simulink model "cl_PWM"  (R2023a)
settings: Solver=FixedStepDiscrete  StartTime=0.0  StopTime=.35  FixedStep=Ts  RelTol=1e-3  EnableMultiTasking=on
PreLoadFcn:
  | ee_ipmsm_velocity_control_data;
StopFcn:
  | ee_addSimlogTimeStamp(bdroot)
values from neighbouring files (symbols this model uses):
  ActCV = 1    [cl_PWM_Parameter.m]
  ActFF = 0    [cl_PWM_Parameter.m]
  down1 = den(1)    [cl_PWM_Parameter.m]
  down2 = den(2)    [cl_PWM_Parameter.m]
  Jm = 7.0616e-06    [cl_PWM_Parameter.m]
  Ki_iq = Ki_id    (= 173.2)    [cl_PWM_Parameter.m]
  Kp_id = 0.6*Tl/Vs/sigma    (= 0.0866)    [cl_PWM_Parameter.m]
  Kp_iq = Kp_id    (= 0.0866)    [cl_PWM_Parameter.m]
  Ld = 0.2e-3    (= 0.0002)    [cl_PWM_Parameter.m]
  Lq = 0.2e-3    (= 0.0002)    [cl_PWM_Parameter.m]
  p = 4    [cl_PWM_Parameter.m]
  psim = 0.0064    [cl_PWM_Parameter.m]
  Trated = 0.2724    [cl_PWM_Parameter.m]
  Ts = 1e-6    (= 1e-06)    [cl_PWM_Parameter.m]
  Tsi = 1/fsw/2    (= 0.0001)    [cl_PWM_Parameter.m]
  Tso = 2*Tsi    (= 0.0002)    [cl_PWM_Parameter.m]
  up = num(2)    [cl_PWM_Parameter.m]
  Vnom = 24    [cl_PWM_Parameter.m]
undefined symbols (not defined in the file or in its folder): denZC_id, denZC_iq, ee_sli_rtmsupport, gcbh, numZC_id, numZC_iq
libraries: nesl_utility x15, fl_lib x10, slpidlib x9, ee_lib x7, spsMeanLib x6, simulink x3, eeTransforms x2, SignalEditorBlockLib x1, eePwmGeneratorTwoLevel x1, slctrlblks x1
(part 1 of 2)
CloseFcn:
  | try,close(h1_ee_ipmsm_velocity_control),end
  | clear h1_ee_ipmsm_velocity_control
  | 
  | clear simlog_ee_ipmsm_velocity_control
  | clear logsout_ee_ipmsm_velocity_control
  | 
  | clear Pmax Tmax p psim Ld Lq L0 Rs Jm
  | clear Cdc Vnom V1 AH0
  | clear Ts fsw Tsi Tso Kp_id Ki_id Kp_iq Ki_iq
  | clear numd_id dend_id numd_iq dend_iq
  | clear Kp_omega Ki_omega numd_omega dend_omega
  | clear ID_MAP IQ_MAP RPM_VECT TQ_VECT VDC_VECT
Description:
  | IPMSM Velocity Control
settings Model: SimulationMode=accelerator  Creator=The MathWorks, Inc.  LastModifiedBy=zxzhu
settings SolverCC: AlgebraicLoopSolver=TrustRegion  AutoInsertRateTranBlk=on  MaxZcPerStep=1
settings DataIOCC: MaxDataPoints=210000  ReturnWorkspaceOutputs=off  SignalLoggingName=logsout_ee_ipmsm_velocity_control
settings OptimizationCC: ReuseModelBlockBuffer=off  LifeSpan=inf
settings DebuggingCC: UnderspecifiedInitializationDetection=Classic  MergeDetectMultiDrivingBlocksExec=none  UnconnectedInputMsg=warning  UnconnectedOutputMsg=warning  UnconnectedLineMsg=warning  SFUnexpectedBacktrackingDiag=warning  SFNoUnconditionalDefaultTransitionDiag=warning  SFExecutionAtInitializationDiag=none  ArithmeticOperatorsInVariantConditions=warning
settings ModelReferenceCC: EnableRefExpFcnMdlSchedulingChecks=on
settings SFSimCC: SimUseLocalCustomCode=off  CustomCodeUndefinedFunction=UseInterfaceOnly
settings RTWCC: RTWUseLocalCustomCode=off  DLArmComputeVersion=19.05
settings CodeAppCC: StateflowObjectComments=on
settings GRTTargetCC: TargetLangStandard=C89/C90 (ANSI)
settings ConfigComp: CovMetricSettings=dw  CovSaveCumulativeToWorkspaceVar=on  CovSaveSingleToWorkspaceVar=on  CovExternalEMLEnable=off
settings SimscapeCC: SimscapeNormalizeSystem=off  SimscapeLogType=all  SimscapeLogSimulationStatistics=on  SimscapeLogName=simlog_ee_ipmsm_velocity_control  SimscapeLogDataHistory=210000

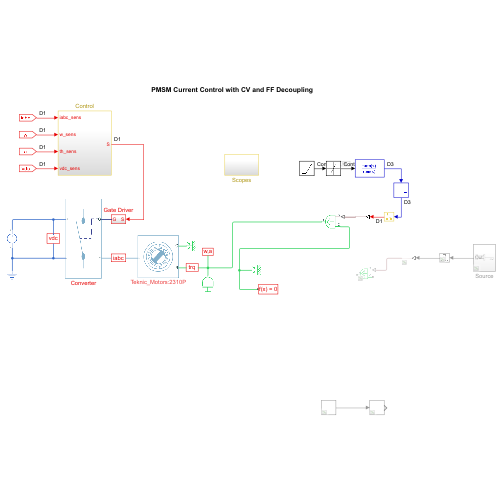
[thumbnail: Simulink's stored preview of the top-level diagram]
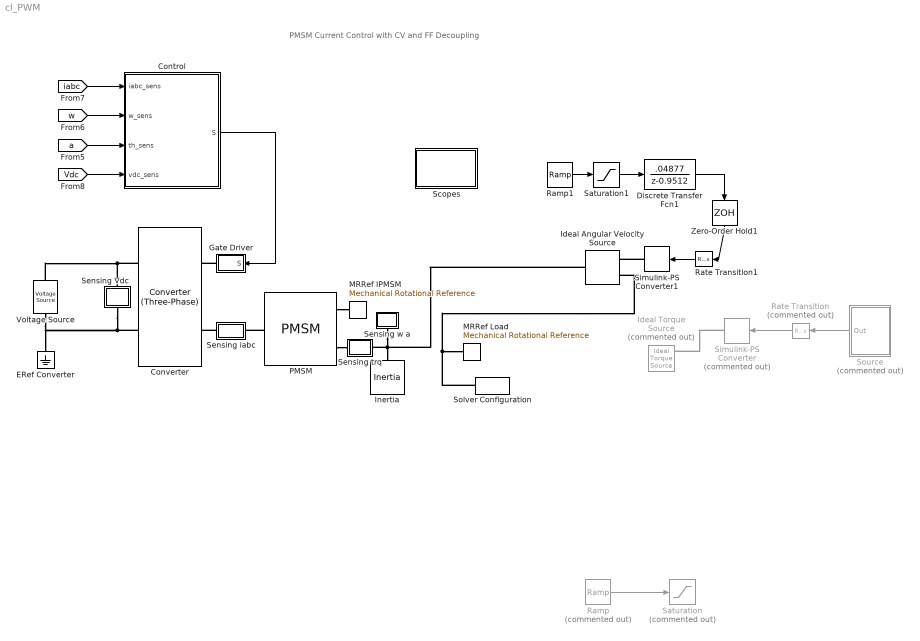
== system cl_PWM ==
  note: PMSM Current Control with CV and FF Decoupling
  Control : Subsystem
  Converter : ee_lib/Semiconductors & Converters/Converters/Converter (Three-Phase)  port_option=ee.enum.threePhasePort.composite  device_type=ee.enum.converters.switchingdevice.mosfet  K=0  Vf=0.8 V  Ron=0.001 Ohm  Rds=0.001 Ohm  Goff=1e-5 1/Ohm  Vgt=1 V  Vgt_off=-1 V  Ih=1 A  Vth=0.5 V  diode_param=2  diode_Vf=0.8 V  diode_Ron=0.001 Ohm  diode_Goff=1e-5 1/Ohm  diode_C=50 nF  diode_iRM=-235 A  diode_iF=300 A  diode_idot=-50 A/us  diode_trr_param=1  diode_trr_factor=3  diode_trr=15 us  diode_Qrr=1.5e+3 s*uA  snubber_type=ee.enum.converters.snubber.include  Cs=1e-7 F  Rs=0.1 Ohm
  Discrete Transfer Fcn1 : DiscreteTransferFcn  Numerator=[.04877]  Denominator=[1 -0.9512]  SampleTime=Tsi
  ERef Converter : fl_lib/Electrical/Electrical Elements/Electrical Reference
  Gate Driver : Subsystem
  Ideal Angular Velocity Source : fl_lib/Mechanical/Mechanical Sources/Ideal Angular Velocity Source
  Ideal Torque Source : fl_lib/Mechanical/Mechanical Sources/Ideal Torque Source  Commented=on
  Inertia : fl_lib/Mechanical/Rotational Elements/Inertia  inertia=Jm kg*m^2  num_ports=foundation.enum.numPorts2.one  w_specify=on  w_priority=High  w=0 rpm  w_nominal_specify=off  w_nominal_unit=rad/s  w_nominal_value=1  t_specify=off  t_priority=High  t=0 N*m  t_nominal_specify=off  t_nominal_unit=N*m  t_nominal_value=1
  MRRef IPMSM : fl_lib/Mechanical/Rotational Elements/Mechanical Rotational Reference
  MRRef Load : fl_lib/Mechanical/Rotational Elements/Mechanical Rotational Reference
  PMSM : ee_lib/Electromechanical/Permanent Magnet/PMSM  Tag={'toolbox/physmod/elec/library/m/ee_lib_parts';'Electromechanical/Permanent_Magnet/PMSM/Teknic_Motors/x2310P.xml'}  port_option=ee.enum.threePhasePort.composite  winding_type=ee.enum.statorconnection.wye  machine_param=ee.enum.pmsm.parameterization.constant  nPolePairs=p  pmflux_param=ee.enum.pmflux.fluxlinkage  pm_flux_linkage=psim Wb  torque_constant=0.0255816607475711 N*m/A  back_emf_constant=0.0255816607475711 V/(rad/s)  stator_param=ee.enum.statorparam.LdLqL0  Ld=Ld H  Lq=Lq H  idVec=[-200 0 200] % Parameter not set A  iqVec=[-200 0 200] % Parameter not set A  LdMatrix=[0.0002 0.0002 0.0002;0.0002 0.0002 0.0002;0.0002 0.0002 0.0002] % Parameter not set H  LqMatrix=[0.0002 0.0002 0.0002;0.0002 0.0002 0.0002;0.0002 0.0002 0.0002] % Parameter not set H  PmMatrix=[0.1 0.1 0.1;0.1 0.1 0.1;0.1 0.1 0.1] Wb  ktMatrix=[0.18 0.18 0.18;0.18 0.18 0.18;0.18 0.18 0.18] N*m/A  keMatrix=[0.18 0.18 0.18;0.18 0.18 0.18;0.18 0.18 0.18] % Parameter not set V/(rad/s)  L0=[] % Parameter not set H  Ls=0.0002 H  Lm=-2e-05 H  Ms=2e-05 H  Rs=Rs Ohm  zero_sequence=ee.enum.park.zerosequence.exclude  axes_param=ee.enum.rotorangle.daxis  loss_param=ee.enum.ironloss.none  losses_oc=[0 0 0] % Parameter not set W  losses_sc=[0 0 0] % Parameter not set W  f_losses=60 % Parameter not set Hz  Isc_losses=95 % Parameter not set A  J=Jm kg*m^2  lam=Trated*.01/3000*9.55 N*m/(rad/s)  i_d_specify=off  i_d_priority=None  i_d=0 A  i_d_nominal_specify=off  i_d_nominal_unit=A  i_d_nominal_value=1  i_q_specify=off  i_q_priority=None  i_q=0 A  i_q_nominal_specify=off  i_q_nominal_unit=A  i_q_nominal_value=1  torque_specify=off  torque_priority=None  torque=0 N*m  torque_nominal_specify=off  torque_nominal_unit=N*m  torque_nominal_value=1  angular_velocity_specify=off  angular_velocity_priority=None  angular_velocity=0 rpm  angular_velocity_nominal_specify=off  angular_velocity_nominal_unit=rpm  angular_velocity_nominal_value=1  angular_position_specify=off  angular_position_priority=High  angular_position=0 rad  angular_position_nominal_specify=off  angular_position_nominal_unit=deg  angular_position_nominal_value=1  alpha=3.93e-3 1/K  alpha_flux=-0.001 1/K  Tmeas=298.15 K  stator_thermal_mass=100 J/K  rotor_thermal_mass=200 J/K  Rm_percent_rotor=90  Rd_percent_rotor=30  temperatureA_specify=off  temperatureA_priority=High  temperatureA=25 degC  temperatureA_nominal_specify=off  temperatureA_nominal_unit=degC  temperatureA_nominal_value=1  temperatureB_specify=off  temperatureB_priority=High  temperatureB=25 degC  temperatureB_nominal_specify=off  temperatureB_nominal_unit=degC  temperatureB_nominal_value=1  temperatureC_specify=off  temperatureC_priority=High  temperatureC=25 degC  temperatureC_nominal_specify=off  temperatureC_nominal_unit=degC  temperatureC_nominal_value=1  temperatureR_specify=off  temperatureR_priority=High  temperatureR=25 degC  temperatureR_nominal_specify=off  temperatureR_nominal_unit=degC  temperatureR_nominal_value=1
      settings: AttributesFormatString=Teknic_Motors:2310P  InternalSimscapePortConfiguration="{\"Bottom\":[],\"Left\":[{\"id\":\"N\",\"label\":\"~\",\"type\":\"foundation.electrical.three_phase\"}],\"Right\":[{\"id\":\"R\",\"label\":\"R\",\"type\":\"foundation.mechanical.rotational.rotational\"},{\"id\":\"C\",\"label\":\"C\",\"type\":\"foundation.mechanical.rotational.rotational\"}],\"Top\":[]}"
  Ramp : simulink/Sources/Ramp  Commented=on  slope=-Trated/.001  start=.25  InitialOutput=0
  Ramp1 : simulink/Sources/Ramp  slope=-3000/9.55/.1  start=0  InitialOutput=0
  Rate Transition : RateTransition  Commented=on  OutPortSampleTime=Ts
  Rate Transition1 : RateTransition  OutPortSampleTime=Ts
  Saturation : Saturate  Commented=on  UpperLimit=.5*Trated  LowerLimit=-.5*Trated
  Saturation1 : Saturate  UpperLimit=3000/9.55*1  LowerLimit=-4800/9.55*1
  Scopes : Subsystem
  Sensing Vdc : Subsystem
      mask Display: disp('vdc')
  Sensing trq : Subsystem
      mask Display: disp('trq')
  Sensing w a : Subsystem
      mask Display: disp('w,a')
  Sensing iabc : Subsystem
      mask Display: disp('iabc')
  Simulink-PS Converter : nesl_utility/Simulink-PS Converter  Commented=on  PhysicalDomain=network_engine_domain  SubClassName=ps_input  LeftPortType=input  RightPortType=output  PseudoPeriodic=off  Frequencies=[]  NoiseDistribution=none  NoiseParameters=[]  Unit=N*m  AffineConversion=off  FilteringAndDerivatives=zero  SimscapeFilterOrder=1  InputFilterTimeConstant=0.001  UdotUserProvided=1
  Simulink-PS Converter1 : nesl_utility/Simulink-PS Converter  PhysicalDomain=network_engine_domain  SubClassName=ps_input  LeftPortType=input  RightPortType=output  PseudoPeriodic=off  Frequencies=[]  NoiseDistribution=none  NoiseParameters=[]  Unit=rad/s  AffineConversion=off  FilteringAndDerivatives=zero  SimscapeFilterOrder=1  InputFilterTimeConstant=0.001  UdotUserProvided=1
  Solver Configuration : nesl_utility/Solver Configuration  PhysicalDomain=network_engine_domain  SubClassName=solver  LeftPortType=input  RightPortType=generic  Tones=[]  Harmonics=[]  SimulateNoise=off  Profile=off  UseLocalSampling=off  EnableSwitchedLinearOptims=on  FrequencyDomain=off  UseCCode=off  RelTol=0.001  AbsTol=1e-06  MinStep=1e-09  ToWorkspace=off  RevertToSquareIcSolve=off  NumHomotopyIterations=100  PhasorMode=off  PhasorModeNumHarmonics=1  ConsistencySolver=NEWTON_FTOL  IndexReductionMethod=DerivativeReplacement  DoDC=off  ResidualTolerance=1e-9  ConsistencyTolSource=GLOBAL  ConsistencyAbsTol=0.001  ConsistencyRelTol=0.001  ConsistencyTolFactor=0.001  UseLocalSolver=on  LocalSolverChoice=NE_BACKWARD_EULER_ADVANCER  ResolveIndetEquations=on  FunctionEvalNumThread=1  LocalSolverSampleTime=Ts  DoFixedCost=on  MaxNonlinIter=5  MaxModeIter=2  ComputeImpulses=off  ImpulseIterations=2  LinearAlgebra=auto  LinearAlgebraNumThread=0  EquationFormulation=NE_TIME_EF  DelaysMemoryBudget=1024  AutomaticFiltering=on  FilteringTimeConstant=0.001  PartitionStorageMethod=AS_NEEDED  PartitionMemoryBudget=1024  PartitionMethod=FAST
  Source : Subsystem  Commented=on
  Voltage Source : ee_lib/Sources/Voltage Source  dc_voltage=Vnom V  ac_voltage=0 V  ac_shift=0 rad  ac_frequency=60 Hz  noise_mode=ee.enum.sources.noise.Disabled  PSD=0 V^2/Hz  sample_time=1e-3 s  repeatability=ee.enum.sources.repeatability.NotRepeatable  user_seed=0  auto_seed=3499211588  i_specify=off  i_priority=None  i=0 A  i_nominal_specify=off  i_nominal_unit=A  i_nominal_value=1  v_specify=off  v_priority=None  v=0 V  v_nominal_specify=off  v_nominal_unit=V  v_nominal_value=1
  Zero-Order Hold1 : ZeroOrderHold  SampleTime=-1
  wires:
  Control/1(S) -> Gate Driver/1(S)
  [Vdc] -> Control/4(vdc_sens)
  [iabc] -> Control/1(iabc_sens)
  [w] -> Control/2(w_sens)
  [a] -> Control/3(th_sens)
  Zero-Order Hold1/1 -> Rate Transition1/1
  Discrete Transfer Fcn1/1 -> Zero-Order Hold1/1
  Ramp1/1 -> Saturation1/1
  Saturation1/1 -> Discrete Transfer Fcn1/1
  Rate Transition1/1 -> Simulink-PS Converter1/1
  Ramp/1 -> Saturation/1
  Source/1(Out) -> Rate Transition/1
  Rate Transition/1 -> Simulink-PS Converter/1
  connections:
  Converter/RConn1 -- Voltage Source/LConn1 -- Sensing Vdc/LConn1
  Inertia/LConn1 -- Ideal Angular Velocity Source/LConn1 -- Sensing w a/LConn1 -- Sensing trq/RConn1
  Gate Driver/RConn1 -- Converter/LConn1
  Solver Configuration/RConn1 -- Ideal Angular Velocity Source/RConn2 -- MRRef Load/LConn1
  Sensing iabc/LConn1 -- Converter/LConn2
  PMSM/RConn2 -- MRRef IPMSM/LConn1
  PMSM/RConn1 -- Sensing trq/LConn1
  Voltage Source/RConn1 -- ERef Converter/LConn1 -- Converter/RConn2 -- Sensing Vdc/RConn1
  PMSM/LConn1 -- Sensing iabc/RConn1
  Simulink-PS Converter1/RConn1 -- Ideal Angular Velocity Source/RConn1
  Simulink-PS Converter/RConn1 -- Ideal Torque Source/RConn1

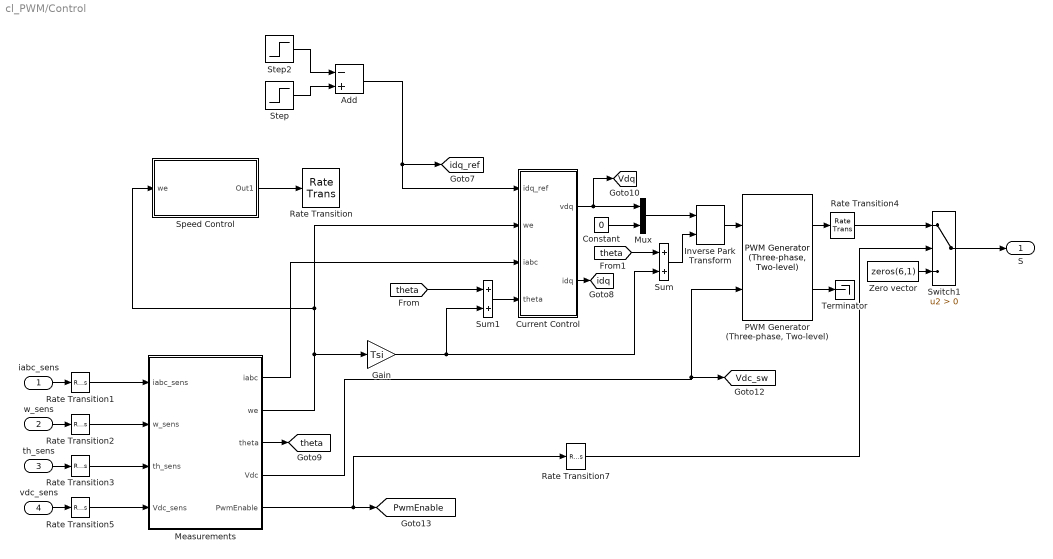
== system cl_PWM/Control ==
  iabc_sens : Inport
  w_sens : Inport  Port=2
  th_sens : Inport  Port=3
  vdc_sens : Inport  Port=4
  Add : Sum  Inputs=-+
  Constant : Constant  Value=0  SampleTime=Tsi
  Current Control : Subsystem
  Gain : Gain  Gain=Tsi
  Inverse Park Transform : eeTransforms/Inverse Park Transform  AxisAlignment=D-axis  PowerInvariant=off
  Measurements : Subsystem
  Mux : Mux  Inputs=2
  "PWM Generator (Three-phase, Two-level)" : eePwmGeneratorTwoLevel/PWM Generator (Three-phase, Two-level)  PWMMode=Continuous PWM (CPWM)  CPWMMode=SVM: space vector modulation  DPWMMode=60 DPWM: 60 degree discontinuous PWM  fsw=fsw  Ts=Ts
      settings: SamplingMode=Asymmetric
  Rate Transition : RateTransition  OutPortSampleTime=Tsi
  Rate Transition{1..3,5,7} (5 alike) : RateTransition
  Rate Transition4 : RateTransition  OutPortSampleTime=Ts
  Speed Control : Subsystem
  Step : Step  Time=.2  Before=[0 0]  After=[0 0.71]  SampleTime=Tsi
  Step2 : Step  Time=.25  Before=[0 0]  After=[0 0.3]  SampleTime=Tsi
  Sum : Sum
  Sum1 : Sum
  Switch1 : Switch  Criteria=u2 > Threshold  SaturateOnIntegerOverflow=off  InputSameDT=off
  Terminator : Terminator
  Zero vector : Constant  Value=zeros(6,1)
  S : Outport  VectorParamsAs1DForOutWhenUnconnected=off
  tag scope: PwmEnable=global, Vdc_sw=global, Vdq=global, idq=global, idq_ref=global, theta=global
  wires:
  Current Control/1(vdq) -> Mux/1, [Vdq]
  Measurements/1(iabc) -> Current Control/3(iabc)
  "PWM Generator (Three-phase, Two-level)"/1 -> Rate Transition4/1
  iabc_sens/1 -> Rate Transition1/1
  w_sens/1 -> Rate Transition2/1
  th_sens/1 -> Rate Transition3/1
  vdc_sens/1 -> Rate Transition5/1
  "PWM Generator (Three-phase, Two-level)"/2 -> Terminator/1
  Rate Transition1/1 -> Measurements/1(iabc_sens)
  Rate Transition2/1 -> Measurements/2(w_sens)
  Rate Transition3/1 -> Measurements/3(th_sens)
  Rate Transition5/1 -> Measurements/4(Vdc_sens)
  Measurements/4(Vdc) -> "PWM Generator (Three-phase, Two-level)"/2, [Vdc_sw]
  Measurements/2(we) -> Gain/1, Speed Control/1(we), Current Control/2(we)
  Current Control/2(idq) -> [idq]
  Switch1/1 -> S/1
  Rate Transition4/1 -> Switch1/1
  Measurements/5(PwmEnable) -> Rate Transition7/1, [PwmEnable]
  Zero vector/1 -> Switch1/3
  Rate Transition7/1 -> Switch1/2
  Constant/1 -> Mux/2
  Inverse Park Transform/1 -> "PWM Generator (Three-phase, Two-level)"/1
  Mux/1 -> Inverse Park Transform/1
  Measurements/3(theta) -> [theta]
  [theta] -> Sum/1
  Sum/1 -> Inverse Park Transform/2
  Gain/1 -> Sum1/2, Sum/2
  Sum1/1 -> Current Control/4(theta)
  [theta] -> Sum1/1
  Speed Control/1(Out1) -> Rate Transition/1
  Step2/1 -> Add/1
  Step/1 -> Add/2
  Add/1 -> Current Control/1(idq_ref), [idq_ref]

== system cl_PWM/Gate Driver ==
  S : Inport
  Demux : Demux  Outputs=6
  Simulink-PS Converter{1..6} (6 alike) : nesl_utility/Simulink-PS Converter  PhysicalDomain=network_engine_domain  SubClassName=ps_input  LeftPortType=input  RightPortType=output  PseudoPeriodic=off  Frequencies=[]  NoiseDistribution=none  NoiseParameters=[]  Unit=1  AffineConversion=off  FilteringAndDerivatives=zero  SimscapeFilterOrder=1  InputFilterTimeConstant=0.001  UdotUserProvided=1
  Six-Pulse Gate Multiplexer : ee_lib/Semiconductors & Converters/Converters/Six-Pulse Gate Multiplexer  port_option=ee.enum.controlport.ps
  G : PMIOPort  Side=Right
  wires:
  Demux/1 -> Simulink-PS Converter1/1
  S/1 -> Demux/1
  Demux/4 -> Simulink-PS Converter4/1
  Demux/2 -> Simulink-PS Converter2/1
  Demux/3 -> Simulink-PS Converter3/1
  Demux/5 -> Simulink-PS Converter5/1
  Demux/6 -> Simulink-PS Converter6/1
  connections:
  Six-Pulse Gate Multiplexer/RConn1 -- G/RConn1
  Simulink-PS Converter1/RConn1 -- Six-Pulse Gate Multiplexer/LConn1
  Simulink-PS Converter3/RConn1 -- Six-Pulse Gate Multiplexer/LConn3
  Simulink-PS Converter5/RConn1 -- Six-Pulse Gate Multiplexer/LConn5
  Simulink-PS Converter6/RConn1 -- Six-Pulse Gate Multiplexer/LConn6
  Simulink-PS Converter4/RConn1 -- Six-Pulse Gate Multiplexer/LConn4
  Simulink-PS Converter2/RConn1 -- Six-Pulse Gate Multiplexer/LConn2

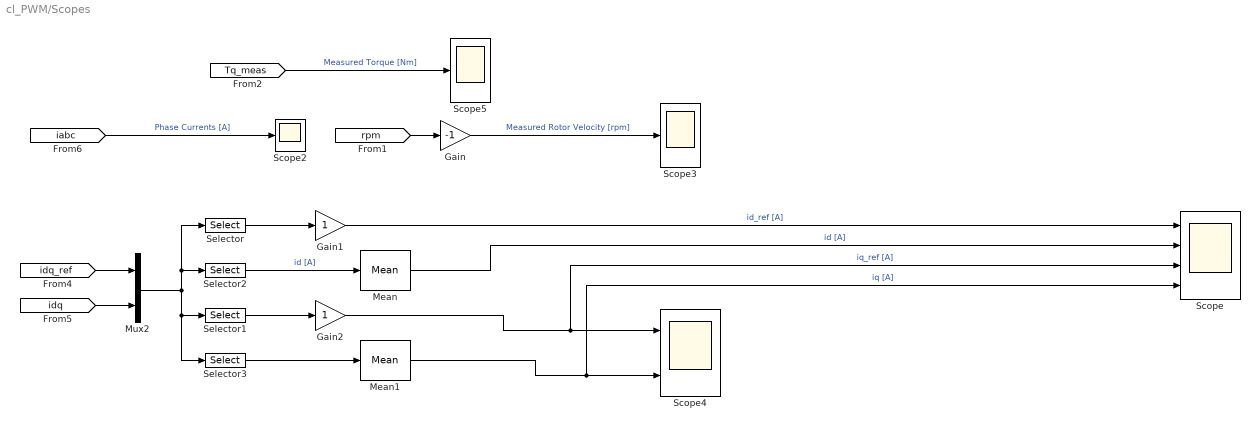
== system cl_PWM/Scopes ==
  Gain : Gain  Gain=-1
  Gain1 : Gain
  Gain2 : Gain
  Mean : spsMeanLib/Mean  Freq=1/Tsi  Vinit=0  Ts=Ts
  Mean1 : spsMeanLib/Mean  Freq=1/Tsi  Vinit=0  Ts=Ts
  Mux2 : Mux  Inputs=2
  Scope : Scope  NumInputPorts=4
  Scope2 : Scope
  Scope3 : Scope
  Scope4 : Scope  NumInputPorts=2
  Scope5 : Scope
  Selector : Selector  InputPortWidth=4  IndexOptions=Index vector (dialog)  Indices=1  OutputSizes=1
  Selector1 : Selector  InputPortWidth=4  IndexOptions=Index vector (dialog)  Indices=2  OutputSizes=1
  Selector2 : Selector  InputPortWidth=4  IndexOptions=Index vector (dialog)  Indices=3  OutputSizes=1
  Selector3 : Selector  InputPortWidth=4  IndexOptions=Index vector (dialog)  Indices=4  OutputSizes=1
  wires:
  Mux2/1 -> Selector3/1, Selector1/1, Selector2/1, Selector/1
  [idq_ref] -> Mux2/1
  [iabc] -> Scope2/1  "Phase Currents [A]"
  [idq] -> Mux2/2
  Selector/1 -> Gain1/1
  Selector1/1 -> Gain2/1
  Gain1/1 -> Scope/1  "id_ref [A]"
  Gain2/1 -> Scope/3, Scope4/1  "iq_ref [A]"
  Mean/1 -> Scope/2  "id [A]"
  [Tq_meas] -> Scope5/1  "Measured Torque [Nm]"
  Selector3/1 -> Mean1/1
  Gain/1 -> Scope3/1  "Measured Rotor Velocity [rpm]"
  Selector2/1 -> Mean/1  "id [A]"
  Mean1/1 -> Scope/4, Scope4/2  "iq [A]"
  [rpm] -> Gain/1

== system cl_PWM/Sensing Vdc ==
  PS-Simulink Converter4 : nesl_utility/PS-Simulink Converter  PhysicalDomain=network_engine_domain  SubClassName=ps_output  LeftPortType=input  RightPortType=output  PseudoPeriodic=off  Frequencies=[]  VectorFormat=1-D array  Unit=V  AffineConversion=off
  Voltage Sensor : fl_lib/Electrical/Electrical Sensors/Voltage Sensor
  + : PMIOPort  Side=Left
  - : PMIOPort  Port=2  Side=Right
  tag scope: Vdc=global
  wires:
  PS-Simulink Converter4/1 -> [Vdc]
  connections:
  Voltage Sensor/LConn1 -- +/RConn1
  Voltage Sensor/RConn2 -- -/RConn1
  PS-Simulink Converter4/LConn1 -- Voltage Sensor/RConn1

== system cl_PWM/Sensing trq ==
  PS-Simulink Converter3 : nesl_utility/PS-Simulink Converter  PhysicalDomain=network_engine_domain  SubClassName=ps_output  LeftPortType=input  RightPortType=output  PseudoPeriodic=off  Frequencies=[]  VectorFormat=1-D array  Unit=N*m  AffineConversion=off
  Torque Sensor : fl_lib/Mechanical/Mechanical Sensors/Ideal Torque Sensor
  R : PMIOPort  Side=Left
  C : PMIOPort  Port=2  Side=Right
  tag scope: Tq_meas=global
  wires:
  PS-Simulink Converter3/1 -> [Tq_meas]
  connections:
  Torque Sensor/RConn1 -- C/RConn1
  Torque Sensor/RConn2 -- PS-Simulink Converter3/LConn1
  Torque Sensor/LConn1 -- R/RConn1

== system cl_PWM/Sensing w a ==
  MRRef : fl_lib/Mechanical/Rotational Elements/Mechanical Rotational Reference
  Motion Sensor : fl_lib/Mechanical/Mechanical Sensors/Ideal Rotational Motion Sensor  reference=foundation.enum.MeasurementReference.difference  acceleration_port=false  velocity_port=true  position_port=true  wrap_angle=false  offset=0 rad
  PS-Simulink Converter1 : nesl_utility/PS-Simulink Converter  PhysicalDomain=network_engine_domain  SubClassName=ps_output  LeftPortType=input  RightPortType=output  PseudoPeriodic=off  Frequencies=[]  VectorFormat=1-D array  Unit=rad/s  AffineConversion=off
  PS-Simulink Converter2 : nesl_utility/PS-Simulink Converter  PhysicalDomain=network_engine_domain  SubClassName=ps_output  LeftPortType=input  RightPortType=output  PseudoPeriodic=off  Frequencies=[]  VectorFormat=1-D array  Unit=rad  AffineConversion=off
  Rate Transition : RateTransition  OutPortSampleTime=Ts
  R : PMIOPort  Side=Left
  tag scope: a=global, w=global
  wires:
  PS-Simulink Converter1/1 -> [w]
  PS-Simulink Converter2/1 -> Rate Transition/1
  Rate Transition/1 -> [a]
  connections:
  R/RConn1 -- Motion Sensor/LConn1
  Motion Sensor/RConn2 -- PS-Simulink Converter1/LConn1
  MRRef/LConn1 -- Motion Sensor/RConn1
  PS-Simulink Converter2/LConn1 -- Motion Sensor/RConn3

== system cl_PWM/Sensing iabc ==
  Current Sensor : ee_lib/Sensors & Transducers/Current Sensor (Three-Phase)
  Floating Neutral (Three-Phase) : ee_lib/Connectors & References/Floating Neutral (Three-Phase)  G_parasitic=1e-12 1/Ohm
      settings: InternalSimscapePortConfiguration="{\"Bottom\":[],\"Left\":[{\"id\":\"N\",\"label\":\"~\",\"type\":\"foundation.electrical.three_phase\"}],\"Right\":[],\"Top\":[]}"
  PS-Simulink Converter : nesl_utility/PS-Simulink Converter  PhysicalDomain=network_engine_domain  SubClassName=ps_output  LeftPortType=input  RightPortType=output  PseudoPeriodic=off  Frequencies=[]  VectorFormat=1-D array  Unit=A  AffineConversion=off
  PS-Simulink Converter1 : nesl_utility/PS-Simulink Converter  PhysicalDomain=network_engine_domain  SubClassName=ps_output  LeftPortType=input  RightPortType=output  PseudoPeriodic=off  Frequencies=[]  VectorFormat=1-D array  Unit=V  AffineConversion=off
  Phase Voltage Sensor (Three-Phase) : ee_lib/Sensors & Transducers/Phase Voltage Sensor (Three-Phase)
  1 : PMIOPort  Side=Left
  2 : PMIOPort  Port=2  Side=Right
  tag scope: Vline=global, iabc=global
  wires:
  PS-Simulink Converter/1 -> [iabc]
  PS-Simulink Converter1/1 -> [Vline]
  connections:
  1/RConn1 -- Current Sensor/LConn1 -- Phase Voltage Sensor (Three-Phase)/LConn1
  2/RConn1 -- Current Sensor/RConn2
  Current Sensor/RConn1 -- PS-Simulink Converter/LConn1
  Floating Neutral (Three-Phase)/LConn1 -- Phase Voltage Sensor (Three-Phase)/RConn2
  PS-Simulink Converter1/LConn1 -- Phase Voltage Sensor (Three-Phase)/RConn1

== system cl_PWM/Source ==
  Add2 : Sum  Inputs=-+
  Step2 : Step  Time=.2  After=Trated*0.5  SampleTime=Tsi
  Step3 : Step  Time=.25  After=Trated*0.5  SampleTime=Tsi
  Out : Outport
  wires:
  Step2/1 -> Add2/2
  Step3/1 -> Add2/1
  Add2/1 -> Out/1

== system cl_PWM/Control/Current Control ==
  idq_ref : Inport
  we : Inport  Port=2
  iabc : Inport  Port=3
  theta : Inport  Port=4
  Constant : Constant  Value=0  SampleTime=Tsi
  PMSM Current Controller with Pre-Control and CV Decoupling : Subsystem  Commented=on  AncestorBlock=eePmsmCurrentController/PMSM Current Controller with Pre-Control  LoadFcn=ee_sli_rtmsupport( 'loadfcn', gcbh );  mask(PMSM Current Controller with Pre-Control){Kp_id=Kp_iq, Ki_id=Ki_iq, Kaw_id=1, Kp_iq=Kp_iq, Ki_iq=Ki_iq, Kaw_iq=1, Ts=-1, Tsd=Tsi, AxisPrio=0, ActZC=on, ActFF=on, idVect=[-200, 0, 200], iqVect=[-200, 0, 200], LdMatrix=Ld * ones(3, 3), LqMatrix=Lq * ones(3, 3), psimMatrix=psim * ones(3, 3)}
      mask prompts: Kp_id "physmod:ee:library:comments:control:eePmsmCurrentController:DaxisCurrentProportionalGain_MP"; Ki_id "physmod:ee:library:comments:control:eePmsmCurrentController:DaxisCurrentIntegralGain_MP"; Kaw_id "physmod:ee:library:comments:control:eePmsmCurrentController:DaxisCurrentAntiwindupGain_MP"; Kp_iq "physmod:ee:library:comments:control:eePmsmCurrentController:QaxisCurrentProportionalGain_MP"; Ki_iq "physmod:ee:library:comments:control:eePmsmCurrentController:QaxisCurrentIntegralGain_MP"; Kaw_iq "physmod:ee:library:comments:control:eePmsmCurrentController:QaxisCurrentAntiwindupGain_MP"; Ts "physmod:ee:library:comments:control:eePmsmCurrentController:SampleTime1ForInherited_MP"; Tsd "physmod:ee:library:comments:control:eePmsmCurrentController:DiscretizationSampleTime_MP"; AxisPrio "physmod:ee:library:comments:control:eePmsmCurrentController:AxisPrioritization_MP"; ActZC "physmod:ee:library:comments:control:eePmsmCurrentController:EnableZeroCancellation_MP"; ActFF "physmod:ee:library:comments:control:eePmsmCurrentController:EnablePrecontrolVoltage_MP"; idVect "physmod:ee:library:comments:control:eePmsmCurrentController:DaxisCurrentVectorIdA_MP"; iqVect "physmod:ee:library:comments:control:eePmsmCurrentController:QaxisCurrentVectorIqA_MP"; LdMatrix "physmod:ee:library:comments:control:eePmsmCurrentController:LdMatrixLdidiqH_MP"; LqMatrix "physmod:ee:library:comments:control:eePmsmCurrentController:LqMatrixLqidiqH_MP"; psimMatrix "physmod:ee:library:comments:control:eePmsmCurrentController:PermanentMagnetFluxLinkageMatrixPMidiqWb_MP"
      mask help: physmod:ee:library:comments:control:eePmsmCurrentController:PMSMCurrentControllerWithPreControl_MD
      mask init:
      | [Tsd, numZC_id, denZC_id, numZC_iq, denZC_iq] = ee.mask.initializePmsmCurrentController(ActZC,Ts,Tsd,Kp_id,Ki_id,Kp_iq,Ki_iq);
      | 
      | if length(idVect) < 2            
      | 	error(message('physmod:simscape:compiler:patterns:checks:LengthGreaterThanOrEqual',getString(message('physmod:ee:library:comments:control:eePmsmCurrentController:DaxisCurrentVectorIdA_MP')), '2'));            
      | end
      | if ~all(diff(idVect) > 0)            
      | 	error(message('physmod:simscape:compiler:patterns:checks:StrictlyAscendingVec',getString(message('physmod:ee:library:comments:control:eePmsmCurrentController:DaxisCurrentVectorIdA_MP'))));            
      | end
      | if length(iqVect) < 2            
      | 	error(message('physmod:simscape:compiler:patterns:checks:LengthGreaterThanOrEqual',getString(message('physmod:ee:library:comments:control:eePmsmCurrentController:QaxisCurrentVectorIqA_MP')), '2'));            
      | end
      | if ~all(diff(iqVect) > 0)            
      | 	error(message('physmod:simscape:compiler:patterns:checks:StrictlyAscendingVec',getString(message('physmod:ee:library:comments:control:eePmsmCurrentController:QaxisCurrentVectorIqA_MP'))));            
      | end
      | if ~all(size(LdMatrix) == [length(idVect), length(iqVect)])            
      | 	error(message('physmod:simscape:compiler:patterns:checks:Size2DEqual',getString(message('physmod:ee:library:comments:control:eePmsmCurrentController:LdMatrixLdidiqH_MP')), getString(message('physmod:ee:library:comments:control:eePmsmCurrentController:DaxisCurrentVectorIdA_MP')), getString(message('physmod:ee:library:comments:control:eePmsmCurrentController:QaxisCurrentVectorIqA_MP'))));            
      | end
      | if ~all(size(LqMatrix) == [length(idVect), length(iqVect)])            
      | 	error(message('physmod:simscape:compiler:patterns:checks:Size2DEqual',getString(message('physmod:ee:library:comments:control:eePmsmCurrentController:LqMatrixLqidiqH_MP')), getString(message('physmod:ee:library:comments:control:eePmsmCurrentController:DaxisCurrentVectorIdA_MP')), getString(message('physmod:ee:library:comments:control:eePmsmCurrentController:QaxisCurrentVectorIqA_MP'))));            
      | end
      | if ~all(size(psimMatrix) == [length(idVect), length(iqVect)])            
      | 	error(message('physmod:simscape:compiler:patterns:checks:Size2DEqual',getString(message('physmod:ee:library:comments:control:eePmsmCurrentController:PermanentMagnetFluxLinkageMatrixPMidiqWb_MP')), getString(message('physmod:ee:library:comments:control:eePmsmCurrentController:DaxisCurrentVectorIdA_MP')), getString(message('physmod:ee:library:comments:control:eePmsmCurrentController:QaxisCurrentVectorIqA_MP'))));            
      | end
      settings: CopyFcn=ee_sli_rtmsupport( 'copyfcn', gcbh );  DeleteFcn=ee_sli_rtmsupport( 'deletefcn', gcbh );  ModelCloseFcn=ee_sli_rtmsupport( 'modelclosefcn', gcbh );  PostSaveFcn=ee_sli_rtmsupport( 'postsavefcn', gcbh );  PreCopyFcn=ee_sli_rtmsupport( 'precopyfcn', gcbh );  OpenFcn=ee_sli_rtmsupport( 'openfcn', gcbh );  CloseFcn=ee_sli_rtmsupport( 'closefcn', gcbh );  PreDeleteFcn=ee_sli_rtmsupport( 'predeletefcn', gcbh );
      mask Help: web(nesl_help(gcbh))
      mask Callback Ts: ee.mask.callbackZeroCancellation(gcb);
      mask TypeOptions AxisPrio: d-q Voltage Limiter/AxisPrio
      mask Callback ActZC: ee.mask.callbackZeroCancellation(gcb);
      mask Callback ActFF: ee.mask.callbackPmsmPreControl(gcb);
      mask DialogControl Container3 Prompt: physmod:ee:library:comments:control:eePmsmCurrentController:tab_ControlParameters
      mask DialogControl Kp_id Prompt: D-axis current proportional gain
      mask DialogControl Ki_id Prompt: D-axis current integral gain
      mask DialogControl Kaw_id Prompt: D-axis current anti-windup gain
      mask DialogControl Kp_iq Prompt: Q-axis current proportional gain
      mask DialogControl Ki_iq Prompt: Q-axis current integral gain
      mask DialogControl Kaw_iq Prompt: Q-axis current anti-windup gain
      mask DialogControl Ts Prompt: Sample time (-1 for inherited)
      mask DialogControl Tsd Prompt: Discretization sample time
      mask DialogControl AxisPrio Prompt: Axis prioritization
      mask DialogControl ActZC Prompt: Enable zero cancellation
      mask DialogControl ActFF Prompt: Enable pre-control voltage
      mask DialogControl Container4 Prompt: physmod:ee:library:comments:control:eePmsmCurrentController:tab_PreControlParameters
      mask DialogControl idVect Prompt: D-axis current vector, id (A)
      mask DialogControl iqVect Prompt: Q-axis current vector, iq (A)
      mask DialogControl LdMatrix Prompt: Ld matrix, Ld(id,iq), (H)
      mask DialogControl LqMatrix Prompt: Lq matrix, Lq(id,iq), (H)
      mask DialogControl psimMatrix Prompt: Permanent magnet flux linkage matrix, PM(id,iq), (Wb)
  Park Transform : eeTransforms/Park Transform  AxisAlignment=D-axis  PowerInvariant=off
  Prefilter_4*50us : DiscreteTransferFcn  Numerator=[.2212]  Denominator=[1 -.7788]
  Selector : Selector  InputPortWidth=3  IndexOptions=Index vector (dialog)  Indices=[1 2]  OutputSizes=1
  Subsystem : Subsystem
  vdq : Outport  VectorParamsAs1DForOutWhenUnconnected=off
  idq : Outport  Port=2  VectorParamsAs1DForOutWhenUnconnected=off
  wires:
  iabc/1 -> Park Transform/1
  we/1 -> Subsystem/3(wElectrical)
  theta/1 -> Park Transform/2
  Constant/1 -> Subsystem/4(Reset)
  Subsystem/1(vdqRef) -> vdq/1
  Park Transform/1 -> Selector/1
  Selector/1 -> idq/1, Subsystem/2(idq)
  idq_ref/1 -> Subsystem/1(idqRef)

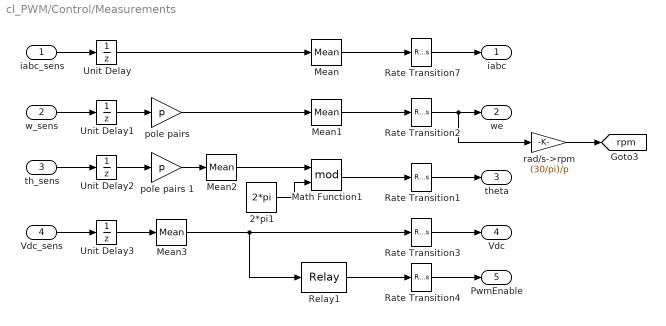
== system cl_PWM/Control/Measurements ==
  iabc_sens : Inport
  w_sens : Inport  Port=2
  th_sens : Inport  Port=3
  Vdc_sens : Inport  Port=4
  2*pi1 : Constant  Value=2*pi  SampleTime=-1
  Math Function1 : Math  Operator=mod  SignedPower=on
  Mean{,1..3} (4 alike) : spsMeanLib/Mean  Freq=1/Tsi  Vinit=0  Ts=Ts
  Rate Transition{1..4,7} (5 alike) : RateTransition  OutPortSampleTime=Tsi
  Relay1 : Relay  OnSwitchValue=.9*Vnom  OffSwitchValue=.8*Vnom
  Unit Delay{,1..3} (4 alike) : UnitDelay  SampleTime=2*Ts  HasFrameUpgradeWarning=on
  pole pairs : Gain  Gain=p
  pole pairs 1 : Gain  Gain=p
  rad/s->rpm : Gain  Gain=(30/pi)/p
  iabc : Outport  VectorParamsAs1DForOutWhenUnconnected=off
  we : Outport  Port=2  VectorParamsAs1DForOutWhenUnconnected=off
  theta : Outport  Port=3  VectorParamsAs1DForOutWhenUnconnected=off
  Vdc : Outport  Port=4  VectorParamsAs1DForOutWhenUnconnected=off
  PwmEnable : Outport  Port=5  VectorParamsAs1DForOutWhenUnconnected=off
  tag scope: rpm=global
  wires:
  Mean2/1 -> Math Function1/1
  Mean1/1 -> Rate Transition2/1
  Mean/1 -> Rate Transition7/1
  Unit Delay1/1 -> pole pairs/1
  Unit Delay3/1 -> Mean3/1
  Unit Delay2/1 -> pole pairs 1/1
  iabc_sens/1 -> Unit Delay/1
  w_sens/1 -> Unit Delay1/1
  Unit Delay/1 -> Mean/1
  Vdc_sens/1 -> Unit Delay3/1
  pole pairs 1/1 -> Mean2/1
  th_sens/1 -> Unit Delay2/1
  pole pairs/1 -> Mean1/1
  Relay1/1 -> Rate Transition4/1
  Mean3/1 -> Rate Transition3/1, Relay1/1
  Math Function1/1 -> Rate Transition1/1
  2*pi1/1 -> Math Function1/2
  Rate Transition7/1 -> iabc/1
  Rate Transition1/1 -> theta/1
  Rate Transition2/1 -> rad/s->rpm/1, we/1
  Rate Transition3/1 -> Vdc/1
  Rate Transition4/1 -> PwmEnable/1
  rad/s->rpm/1 -> [rpm]

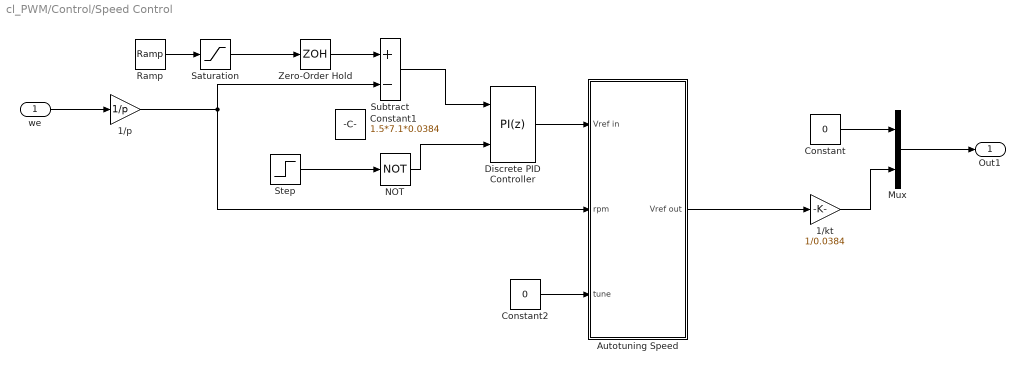
== system cl_PWM/Control/Speed Control ==
  we : Inport
  1/kt : Gain  Gain=1/0.0384
  1/p : Gain  Gain=1/p
  Autotuning Speed : Subsystem
  Constant : Constant  Value=0
  Constant1 : Constant  Value=1.5*7.1*0.0384  SampleTime=Tso
  Constant2 : Constant  Value=0  SampleTime=Tso
  Discrete PID Controller : slpidlib/PID Controller  Controller=PI  Form=Parallel  TimeDomain=Discrete-time  UseExternalTs=off  SampleTime=-1  IntegratorMethod=Forward Euler  FilterMethod=Forward Euler  ControllerParametersSource=internal  P=.04565*0.2  I=9.021*0.1  UseKiTs=off  D=0  N=100  UseFilter=on  TunerSelectOption=Transfer Function Based (PID Tuner App)  InitialConditionSource=internal  InitialConditionForIntegrator=0  InitialConditionForFilter=0  DifferentiatorICPrevScaledInput=0  ExternalReset=level  TrackingMode=off  Kt=1  LimitOutput=on  SatLimitsSource=internal  UpperSaturationLimit=1.5*Trated  LowerSaturationLimit=-1.5*Trated  LinearizeAsGain=off  AntiWindupMode=clamping  Kb=1  LimitIntegrator=on  UpperIntegratorSaturationLimit=1.5*Trated*.9  LowerIntegratorSaturationLimit=-1.5*Trated*.9  POutMin=[]  POutMax=[]  IOutMin=[]  IOutMax=[]  DOutMin=[]  DOutMax=[]  NOutMin=[]  NOutMax=[]  SumOutMin=[]  SumOutMax=[]  SaturationOutMin=[]  SaturationOutMax=[]  PParamMin=[]  PParamMax=[]  IParamMin=[]  IParamMax=[]  DParamMin=[]  DParamMax=[]  NParamMin=[]  NParamMax=[]  KbParamMin=[]  KbParamMax=[]  KtParamMin=[]  KtParamMax=[]  KbOutMin=[]  KbOutMax=[]  KtOutMin=[]  KtOutMax=[]  IntegratorOutMin=[]  IntegratorOutMax=[]  FilterOutMin=[]  FilterOutMax=[]  SumI1OutMin=[]  SumI1OutMax=[]  SumI2OutMin=[]  SumI2OutMax=[]  SumI3OutMin=[]  SumI3OutMax=[]  SumI4OutMin=[]  SumI4OutMax=[]  SumDOutMin=[]  SumDOutMax=[]  DifferentiatorOutMin=[]  DifferentiatorOutMax=[]  FilterDiffOutCoefMin=[]  FilterDiffOutCoefMax=[]  ReciprocalOutMin=[]  ReciprocalOutMax=[]  SumDenOutMin=[]  SumDenOutMax=[]  SumNumOutMin=[]  SumNumOutMax=[]  DivideOutMin=[]  DivideOutMax=[]  UdiffTsProdOutMin=[]  UdiffTsProdOutMax=[]  NTsProdOutMin=[]  NTsProdOutMax=[]  UintegralTsProdOutMin=[]  UintegralTsProdOutMax=[]  UngainTsProdOutMin=[]  UngainTsProdOutMax=[]  ClampingZeroOutDataTypeStr=Inherit: Inherit via back propagation  ClampingZeroOutMin=[]  ClampingZeroOutMax=[]  FilterDenConstantOutDataTypeStr=Inherit: Inherit via back propagation  FilterDenConstantOutMin=[]  FilterDenConstantOutMax=[]  PCopyOutDataTypeStr=Inherit: Inherit via back propagation  PCopyOutMin=[]  PCopyOutMax=[]  NCopyOutDataTypeStr=Inherit: Inherit via back propagation  NCopyOutMin=[]  NCopyOutMax=[]  IntegratorContinuousStateAttributes=''  IntegratorStateMustResolveToSignalObject=off  IntegratorRTWStateStorageClass=Auto  FilterContinuousStateAttributes=''  FilterStateMustResolveToSignalObject=off  FilterRTWStateStorageClass=Auto  ParallelPVariant=InternalParameters  IdealPVariant=Disabled  IVariant=InternalParameters  DVariant=Disabled  IntegratorVariant=Discrete  SatVariant=Enabled  AWVariant=DiscClampingParallel  PCopyVariant=Disabled  TRVariant=Disabled  FdbkBlocksVariant=Forward  IdealPFdbkVariant=Disabled  SatFdbkVariant=Disabled  DerivativeFilterVariant=Disabled  NVariant=Disabled  NCopyVariant=Disabled_SignalSpec  FilterICVariant=Disabled  IntegratorICVariant=InternalICs  ExternalResetVariant=ExternalReset  TRSumVariant=Passthrough  SumFdbkVariant=Disabled  SumVariant=Sum_PI  TsampFilterVariant=InternalTs  TsampNgainVariant=Passthrough  TsampIntegralVariant=Disabled_SignalSpec  ExternalSaturationOutDataTypeStr=Inherit: Same as second input
      settings: LibrarySourceBlock=|
      | hdlsllib/HDL Floating Point
      | Operations/Discrete PID Controller
  Mux : Mux  Inputs=2
  NOT : Logic  Operator=NOT  IconShape=distinctive  AllPortsSameDT=off  OutDataTypeStr=boolean
  Ramp : simulink/Sources/Ramp  slope=3000/9.55/.1  start=.05  InitialOutput=0
  Saturation : Saturate  UpperLimit=3000/9.55*3/3  LowerLimit=-3000/9.55*1.0
  Step : Step  Time=.01  SampleTime=Tso
  Subtract : Sum  Inputs=+-
  Zero-Order Hold : ZeroOrderHold  SampleTime=Tso
  Out1 : Outport
  wires:
  Ramp/1 -> Saturation/1
  1/p/1 -> Subtract/2, Autotuning Speed/2(rpm)
  Saturation/1 -> Zero-Order Hold/1
  Step/1 -> NOT/1
  we/1 -> 1/p/1
  Discrete PID Controller/1 -> Autotuning Speed/1(Vref in)
  Autotuning Speed/1(Vref out) -> 1/kt/1
  Constant2/1 -> Autotuning Speed/3(tune)
  Constant/1 -> Mux/1
  1/kt/1 -> Mux/2
  Mux/1 -> Out1/1
  Subtract/1 -> Discrete PID Controller/1
  NOT/1 -> Discrete PID Controller/2
  Zero-Order Hold/1 -> Subtract/1

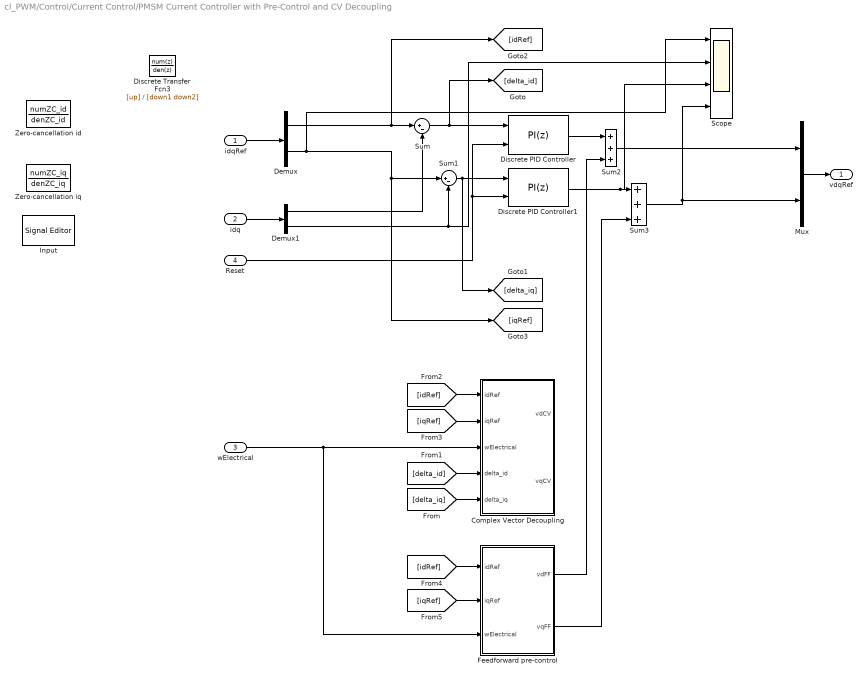
== system cl_PWM/Control/Current Control/PMSM Current Controller with Pre-Control and CV Decoupling ==
  idqRef : Inport  SampleTime=Ts
  idq : Inport  Port=2  SampleTime=Ts
  wElectrical : Inport  Port=3  SampleTime=Ts
  Reset : Inport  Port=4  SampleTime=Ts
  Complex Vector Decoupling : Subsystem
  Demux : Demux  Outputs=2
  Demux1 : Demux  Outputs=2
  Discrete Transfer Fcn3 : DiscreteTransferFcn  Numerator=[up]  Denominator=[down1 down2]
  Discrete PID Controller : slpidlib/PID Controller  Controller=PI  Form=Parallel  TimeDomain=Discrete-time  UseExternalTs=off  SampleTime=Tsi  IntegratorMethod=Forward Euler  FilterMethod=Forward Euler  ControllerParametersSource=internal  P=Kp_id  I=Ki_id  UseKiTs=on  D=0  N=100  UseFilter=on  TunerSelectOption=Transfer Function Based (PID Tuner App)  InitialConditionSource=internal  InitialConditionForIntegrator=0  InitialConditionForFilter=0  DifferentiatorICPrevScaledInput=0  ExternalReset=level  TrackingMode=off  Kt=1  LimitOutput=on  SatLimitsSource=internal  UpperSaturationLimit=Vnom/1.732  LowerSaturationLimit=-Vnom/1.732  LinearizeAsGain=off  AntiWindupMode=clamping  Kb=1  LimitIntegrator=on  UpperIntegratorSaturationLimit=.9*Vnom/1.732  LowerIntegratorSaturationLimit=-.9*Vnom/1.732  POutMin=[]  POutMax=[]  IOutMin=[]  IOutMax=[]  DOutMin=[]  DOutMax=[]  NOutMin=[]  NOutMax=[]  SumOutMin=[]  SumOutMax=[]  SaturationOutMin=[]  SaturationOutMax=[]  PParamMin=[]  PParamMax=[]  IParamMin=[]  IParamMax=[]  DParamMin=[]  DParamMax=[]  NParamMin=[]  NParamMax=[]  KbParamMin=[]  KbParamMax=[]  KtParamMin=[]  KtParamMax=[]  KbOutMin=[]  KbOutMax=[]  KtOutMin=[]  KtOutMax=[]  IntegratorOutMin=[]  IntegratorOutMax=[]  FilterOutMin=[]  FilterOutMax=[]  SumI1OutMin=[]  SumI1OutMax=[]  SumI2OutMin=[]  SumI2OutMax=[]  SumI3OutMin=[]  SumI3OutMax=[]  SumI4OutMin=[]  SumI4OutMax=[]  SumDOutMin=[]  SumDOutMax=[]  DifferentiatorOutMin=[]  DifferentiatorOutMax=[]  FilterDiffOutCoefMin=[]  FilterDiffOutCoefMax=[]  ReciprocalOutMin=[]  ReciprocalOutMax=[]  SumDenOutMin=[]  SumDenOutMax=[]  SumNumOutMin=[]  SumNumOutMax=[]  DivideOutMin=[]  DivideOutMax=[]  UdiffTsProdOutMin=[]  UdiffTsProdOutMax=[]  NTsProdOutMin=[]  NTsProdOutMax=[]  UintegralTsProdOutMin=[]  UintegralTsProdOutMax=[]  UngainTsProdOutMin=[]  UngainTsProdOutMax=[]  ClampingZeroOutDataTypeStr=Inherit: Inherit via back propagation  ClampingZeroOutMin=[]  ClampingZeroOutMax=[]  FilterDenConstantOutDataTypeStr=Inherit: Inherit via back propagation  FilterDenConstantOutMin=[]  FilterDenConstantOutMax=[]  PCopyOutDataTypeStr=Inherit: Inherit via back propagation  PCopyOutMin=[]  PCopyOutMax=[]  NCopyOutDataTypeStr=Inherit: Inherit via back propagation  NCopyOutMin=[]  NCopyOutMax=[]  IntegratorContinuousStateAttributes=''  IntegratorStateMustResolveToSignalObject=off  IntegratorRTWStateStorageClass=Auto  FilterContinuousStateAttributes=''  FilterStateMustResolveToSignalObject=off  FilterRTWStateStorageClass=Auto  ParallelPVariant=InternalParameters  IdealPVariant=Disabled  IVariant=InternalParameters  DVariant=Disabled  IntegratorVariant=Discrete  SatVariant=Enabled  AWVariant=DiscClampingParallel  PCopyVariant=Disabled  TRVariant=Disabled  FdbkBlocksVariant=Forward  IdealPFdbkVariant=Disabled  SatFdbkVariant=Disabled  DerivativeFilterVariant=Disabled  NVariant=Disabled  NCopyVariant=Disabled_SignalSpec  FilterICVariant=Disabled  IntegratorICVariant=InternalICs  ExternalResetVariant=ExternalReset  TRSumVariant=Passthrough  SumFdbkVariant=Disabled  SumVariant=Sum_PI  TsampFilterVariant=InternalTs  TsampNgainVariant=Passthrough  TsampIntegralVariant=Disabled_SignalSpec  ExternalSaturationOutDataTypeStr=Inherit: Same as second input
      settings: LibrarySourceBlock=simulink/Discrete/Discrete PID Controller
  Discrete PID Controller1 : slpidlib/PID Controller  Controller=PI  Form=Parallel  TimeDomain=Discrete-time  UseExternalTs=off  SampleTime=Tsi  IntegratorMethod=Forward Euler  FilterMethod=Forward Euler  ControllerParametersSource=internal  P=Kp_iq  I=Ki_iq  UseKiTs=on  D=0  N=100  UseFilter=on  TunerSelectOption=Transfer Function Based (PID Tuner App)  InitialConditionSource=internal  InitialConditionForIntegrator=0  InitialConditionForFilter=0  DifferentiatorICPrevScaledInput=0  ExternalReset=level  TrackingMode=off  Kt=1  LimitOutput=on  SatLimitsSource=internal  UpperSaturationLimit=Vnom/1.732  LowerSaturationLimit=-Vnom/1.732  LinearizeAsGain=off  AntiWindupMode=clamping  Kb=1  LimitIntegrator=on  UpperIntegratorSaturationLimit=.9*Vnom/1.732  LowerIntegratorSaturationLimit=-.9*Vnom/1.732  POutMin=[]  POutMax=[]  IOutMin=[]  IOutMax=[]  DOutMin=[]  DOutMax=[]  NOutMin=[]  NOutMax=[]  SumOutMin=[]  SumOutMax=[]  SaturationOutMin=[]  SaturationOutMax=[]  PParamMin=[]  PParamMax=[]  IParamMin=[]  IParamMax=[]  DParamMin=[]  DParamMax=[]  NParamMin=[]  NParamMax=[]  KbParamMin=[]  KbParamMax=[]  KtParamMin=[]  KtParamMax=[]  KbOutMin=[]  KbOutMax=[]  KtOutMin=[]  KtOutMax=[]  IntegratorOutMin=[]  IntegratorOutMax=[]  FilterOutMin=[]  FilterOutMax=[]  SumI1OutMin=[]  SumI1OutMax=[]  SumI2OutMin=[]  SumI2OutMax=[]  SumI3OutMin=[]  SumI3OutMax=[]  SumI4OutMin=[]  SumI4OutMax=[]  SumDOutMin=[]  SumDOutMax=[]  DifferentiatorOutMin=[]  DifferentiatorOutMax=[]  FilterDiffOutCoefMin=[]  FilterDiffOutCoefMax=[]  ReciprocalOutMin=[]  ReciprocalOutMax=[]  SumDenOutMin=[]  SumDenOutMax=[]  SumNumOutMin=[]  SumNumOutMax=[]  DivideOutMin=[]  DivideOutMax=[]  UdiffTsProdOutMin=[]  UdiffTsProdOutMax=[]  NTsProdOutMin=[]  NTsProdOutMax=[]  UintegralTsProdOutMin=[]  UintegralTsProdOutMax=[]  UngainTsProdOutMin=[]  UngainTsProdOutMax=[]  ClampingZeroOutDataTypeStr=Inherit: Inherit via back propagation  ClampingZeroOutMin=[]  ClampingZeroOutMax=[]  FilterDenConstantOutDataTypeStr=Inherit: Inherit via back propagation  FilterDenConstantOutMin=[]  FilterDenConstantOutMax=[]  PCopyOutDataTypeStr=Inherit: Inherit via back propagation  PCopyOutMin=[]  PCopyOutMax=[]  NCopyOutDataTypeStr=Inherit: Inherit via back propagation  NCopyOutMin=[]  NCopyOutMax=[]  IntegratorContinuousStateAttributes=''  IntegratorStateMustResolveToSignalObject=off  IntegratorRTWStateStorageClass=Auto  FilterContinuousStateAttributes=''  FilterStateMustResolveToSignalObject=off  FilterRTWStateStorageClass=Auto  ParallelPVariant=InternalParameters  IdealPVariant=Disabled  IVariant=InternalParameters  DVariant=Disabled  IntegratorVariant=Discrete  SatVariant=Enabled  AWVariant=DiscClampingParallel  PCopyVariant=Disabled  TRVariant=Disabled  FdbkBlocksVariant=Forward  IdealPFdbkVariant=Disabled  SatFdbkVariant=Disabled  DerivativeFilterVariant=Disabled  NVariant=Disabled  NCopyVariant=Disabled_SignalSpec  FilterICVariant=Disabled  IntegratorICVariant=InternalICs  ExternalResetVariant=ExternalReset  TRSumVariant=Passthrough  SumFdbkVariant=Disabled  SumVariant=Sum_PI  TsampFilterVariant=InternalTs  TsampNgainVariant=Passthrough  TsampIntegralVariant=Disabled_SignalSpec  ExternalSaturationOutDataTypeStr=Inherit: Same as second input
      settings: LibrarySourceBlock=simulink/Discrete/Discrete PID Controller
  Feedforward pre-control : Subsystem
  Input : SignalEditorBlockLib/Signal Editor  FileName=ee_ipmsm_velocity_control_Input.mat  ActiveScenario=Test_i  ActiveSignal=id_ref  IsBus=off  OutputBusObjectStr=Bus: BusObject  SampleTime=Tsi  Interpolate=off  ZeroCross=off  OutputAfterFinalValue=Setting to zero  Unit=inherit  PreserveSignalName=on  ApplySigPropsToAllScenarios=on
  Mux : Mux  Inputs=2
  Scope : Scope  NumInputPorts=4
  Sum : Sum  Inputs=|+-
  Sum1 : Sum  Inputs=|+-
  Sum2 : Sum  Inputs=+++
  Sum3 : Sum  Inputs=+++
  Zero-cancellation id : DiscreteTransferFcn  Numerator=numZC_id  Denominator=denZC_id  SampleTime=Ts
  Zero-cancellation iq : DiscreteTransferFcn  Numerator=numZC_iq  Denominator=denZC_iq  SampleTime=Ts
  vdqRef : Outport  VectorParamsAs1DForOutWhenUnconnected=off
  wires:
  Reset/1 -> Discrete PID Controller1/2, Discrete PID Controller/2
  idq/1 -> Demux1/1
  Demux1/2 -> Sum1/2, Scope/2
  Demux1/1 -> Sum/2
  Sum/1 -> [delta_id], Discrete PID Controller/1
  Sum1/1 -> [delta_iq], Discrete PID Controller1/1
  Discrete PID Controller/1 -> Sum2/1
  Demux/2 -> Sum1/1, [iqRef], Scope/1
  Discrete PID Controller1/1 -> Scope/3, Sum3/1
  Mux/1 -> vdqRef/1
  Demux/1 -> [idRef], Sum/1
  wElectrical/1 -> Feedforward pre-control/3(wElectrical), Complex Vector Decoupling/3(wElectrical)
  [delta_id] -> Complex Vector Decoupling/4(delta_id)
  [delta_iq] -> Complex Vector Decoupling/5(delta_iq)
  [idRef] -> Complex Vector Decoupling/1(idRef)
  [iqRef] -> Complex Vector Decoupling/2(iqRef)
  [idRef] -> Feedforward pre-control/1(idRef)
  [iqRef] -> Feedforward pre-control/2(iqRef)
  idqRef/1 -> Demux/1
  Feedforward pre-control/2(vqFF) -> Sum3/3
  Feedforward pre-control/1(vdFF) -> Sum2/3
  Sum2/1 -> Mux/1
  Sum3/1 -> Scope/4, Mux/2
